simulink model "magDesat_test_2"  (R2018b)
settings: Solver=FixedStepAuto  StartTime=0.0  StopTime=25000  RelTol=1e-3
undefined symbols (not defined in the file or in its folder): DiscIntNeverNeededParam, fswParams, satelliteDynamics_lib, simParams
libraries: vrlib x2, Desaturation_Controller_lib x1, Detumbling_Controller_lib x1, Environment_lib x1, rwa_assembly_torqueinput_lib x1, aerolibutil x1, sharedutil x1
settings Model: Creator=colem  LastModifiedBy=colem

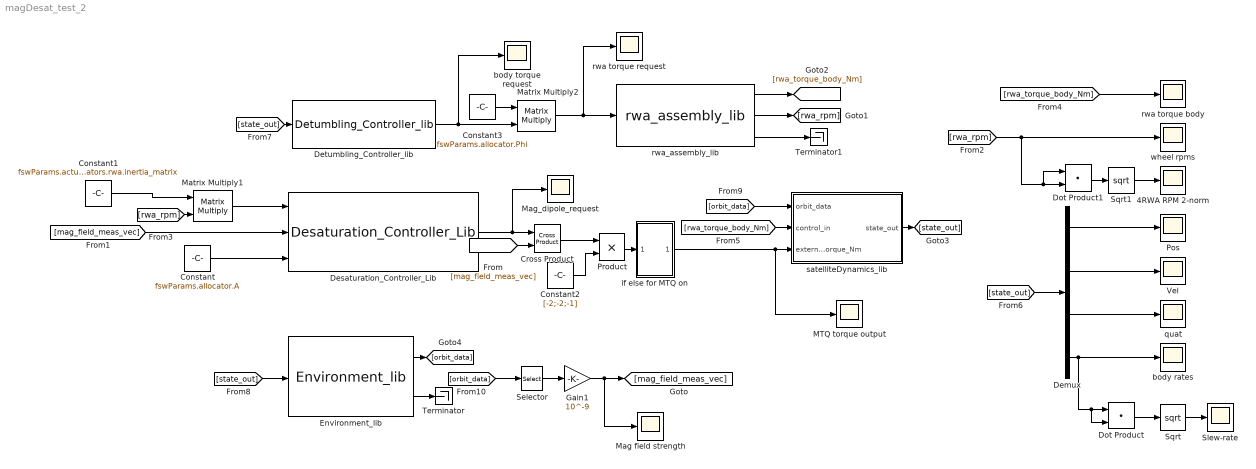
== system magDesat_test_2 ==
  4RWA RPM 2-norm : Scope
  Constant : Constant  Value=fswParams.allocator.A
  Constant1 : Constant  Value=fswParams.actuators.rwa.inertia_matrix
  Constant2 : Constant  Value=[-2;-2;-1]
  Constant3 : Constant  Value=fswParams.allocator.Phi
  Cross Product : vrlib/Utilities/Cross Product
      settings: SourceProductBaseCode=VR
  Demux : Demux  Outputs=[3 3 4 3]
  Desaturation_Controller_Lib : Desaturation_Controller_lib/Desaturation_Controller_Lib  SystemSampleTime=-1
  Detumbling_Controller_lib : Detumbling_Controller_lib/Detumbling_Controller_lib  SystemSampleTime=-1
  Dot Product : DotProduct  InputSameDT=on  OutDataTypeStr=Inherit: Inherit via internal rule
  Dot Product1 : DotProduct  InputSameDT=on  OutDataTypeStr=Inherit: Inherit via internal rule
  Environment_lib : Environment_lib/Environment_lib  SystemSampleTime=-1
  Gain1 : Gain  Gain=10^-9
  MTQ torque output : Scope
  Mag field strength : Scope
  Mag_dipole_request : Scope
  Matrix Multiply1 : Product  Multiplication=Matrix(*)
  Matrix Multiply2 : Product  Multiplication=Matrix(*)
  Pos : Scope
  Product : Product
  Selector : Selector  InputPortWidth=13  IndexOptions=Index vector (dialog)  Indices=[11 12 13]  OutputSizes=1
  Slew-rate : Scope
  Sqrt : Sqrt  SaturateOnIntegerOverflow=on
  Sqrt1 : Sqrt  SaturateOnIntegerOverflow=on
  Terminator : Terminator
  Terminator1 : Terminator
  Vel : Scope
  body rates : Scope
  body torque request : Scope
  if else for MTQ on : Subsystem
  quat : Scope
  rwa torque body : Scope
  rwa torque request : Scope
  rwa_assembly_lib : rwa_assembly_torqueinput_lib/rwa_assembly_lib  SystemSampleTime=-1
  satelliteDynamics_lib : Subsystem  AncestorBlock=satelliteDynamics_lib/satelliteDynamics_lib
  wheel rpms : Scope
  wires:
  Detumbling_Controller_lib/1 -> Matrix Multiply2/2, body torque request/1
  Environment_lib/2 -> Terminator/1
  Desaturation_Controller_Lib/1 -> Mag_dipole_request/1, Cross Product/1
  Constant/1 -> Desaturation_Controller_Lib/3
  Cross Product/1 -> Product/1
  Constant1/1 -> Matrix Multiply1/1
  rwa_assembly_lib/3 -> Terminator1/1
  Matrix Multiply1/1 -> Desaturation_Controller_Lib/1
  Constant3/1 -> Matrix Multiply2/1
  Matrix Multiply2/1 -> rwa_assembly_lib/1, rwa torque request/1
  [mag_field_meas_vec] -> Desaturation_Controller_Lib/2
  [mag_field_meas_vec] -> Cross Product/2
  Product/1 -> if else for MTQ on/1(In1)
  if else for MTQ on/1(Out1) -> MTQ torque output/1, satelliteDynamics_lib/3(external_torque_Nm)
  Selector/1 -> Gain1/1
  Gain1/1 -> Mag field strength/1, [mag_field_meas_vec]
  Dot Product/1 -> Sqrt/1
  Sqrt/1 -> Slew-rate/1
  Sqrt1/1 -> 4RWA RPM 2-norm/1
  Dot Product1/1 -> Sqrt1/1
  Demux/4 -> Dot Product/1, Dot Product/2, body rates/1
  Demux/3 -> quat/1
  Demux/2 -> Vel/1
  Demux/1 -> Pos/1
  Constant2/1 -> Product/2
  [rwa_rpm] -> Matrix Multiply1/2
  rwa_assembly_lib/2 -> [rwa_rpm]
  [rwa_rpm] -> wheel rpms/1, Dot Product1/1, Dot Product1/2
  [rwa_torque_body_Nm] -> satelliteDynamics_lib/2(control_in)
  [rwa_torque_body_Nm] -> rwa torque body/1
  rwa_assembly_lib/1 -> [rwa_torque_body_Nm]
  satelliteDynamics_lib/1(state_out) -> [state_out]
  [state_out] -> Demux/1
  [state_out] -> Environment_lib/1
  [state_out] -> Detumbling_Controller_lib/1
  [orbit_data] -> Selector/1
  [orbit_data] -> satelliteDynamics_lib/1(orbit_data)
  Environment_lib/1 -> [orbit_data]

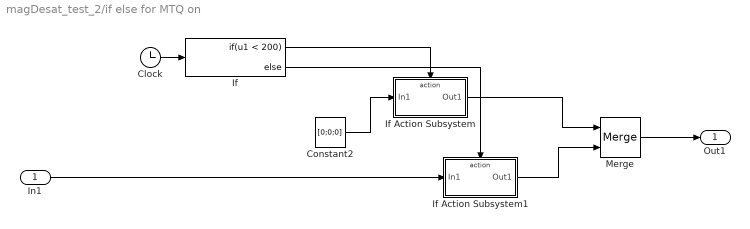
== system magDesat_test_2/if else for MTQ on ==
  In1 : Inport
  Clock : Clock
  Constant2 : Constant  Value=[0;0;0]
  If : If  IfExpression=u1 < 200
  If Action Subsystem : Subsystem  TreatAsAtomicUnit=on
  If Action Subsystem1 : Subsystem  TreatAsAtomicUnit=on
  Merge : Merge
  Out1 : Outport
  wires:
  Clock/1 -> If/1
  If/2 -> If Action Subsystem1/Action
  Constant2/1 -> If Action Subsystem/1(In1)
  Merge/1 -> Out1/1
  If Action Subsystem1/1(Out1) -> Merge/2
  If Action Subsystem/1(Out1) -> Merge/1
  If/1 -> If Action Subsystem/Action
  In1/1 -> If Action Subsystem1/1(In1)

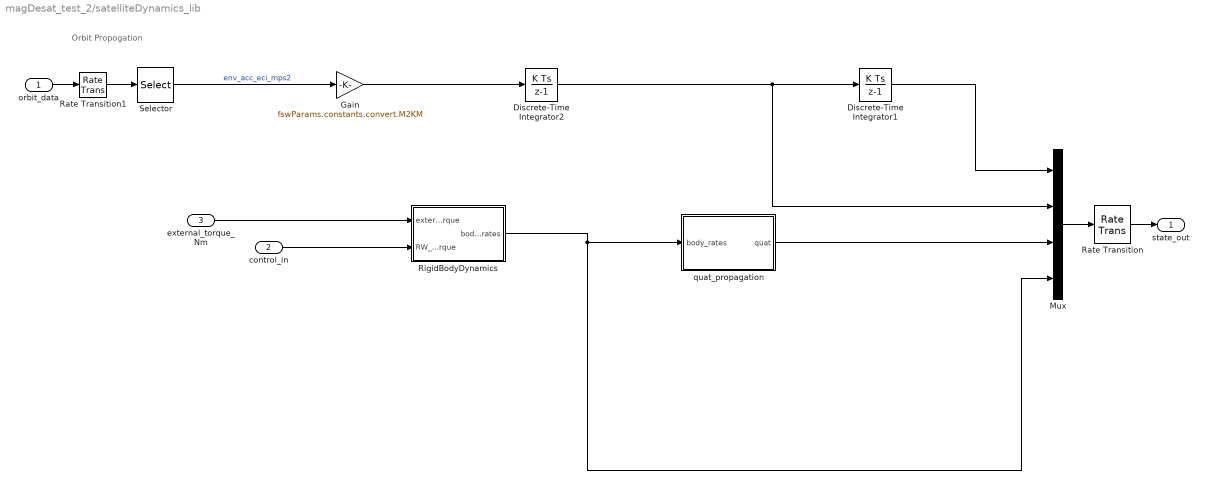
== system magDesat_test_2/satelliteDynamics_lib ==
  note: Orbit Propogation
  orbit_data : Inport
  control_in : Inport  Port=2
  external_torque_Nm : Inport  Port=3
  Discrete-Time Integrator1 : DiscreteIntegrator  InitialCondition=simParams.initialConditions.r0  SampleTime=-1  ICPrevOutput=DiscIntNeverNeededParam  ICPrevScaledInput=DiscIntNeverNeededParam
  Discrete-Time Integrator2 : DiscreteIntegrator  InitialCondition=simParams.initialConditions.v0  SampleTime=-1  ICPrevOutput=DiscIntNeverNeededParam  ICPrevScaledInput=DiscIntNeverNeededParam
  Gain : Gain  Gain=fswParams.constants.convert.M2KM
  Mux : Mux  Inputs=[3 3 4 3]
  Rate Transition : RateTransition  InitialCondition=[simParams.initialConditions.r0;simParams.initialConditions.v0;simParams.initialConditions.q0;simParams.initialConditions.w0]
  Rate Transition1 : RateTransition  OutPortSampleTime=simParams.sample_time_s
  RigidBodyDynamics : Subsystem
  Selector : Selector  InputPortWidth=13  IndexOptions=Index vector (dialog)  Indices=[1 2 3]  OutputSizes=1
  quat_propagation : Subsystem
  state_out : Outport
  wires:
  control_in/1 -> RigidBodyDynamics/2(RW_torque)
  Mux/1 -> Rate Transition/1
  Discrete-Time Integrator2/1 -> Mux/2, Discrete-Time Integrator1/1
  Discrete-Time Integrator1/1 -> Mux/1
  Gain/1 -> Discrete-Time Integrator2/1
  Rate Transition/1 -> state_out/1
  orbit_data/1 -> Rate Transition1/1
  Rate Transition1/1 -> Selector/1
  external_torque_Nm/1 -> RigidBodyDynamics/1(external_torque)
  Selector/1 -> Gain/1  "env_acc_eci_mps2"
  quat_propagation/1(quat) -> Mux/3
  RigidBodyDynamics/1(body_rates) -> Mux/4, quat_propagation/1(body_rates)

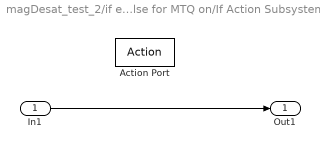
== system magDesat_test_2/if else for MTQ on/If Action Subsystem ==
  In1 : Inport
  Action Port : ActionPort  ActionType=then
  Out1 : Outport
  wires:
  In1/1 -> Out1/1

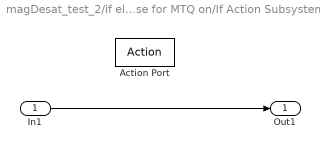
== system magDesat_test_2/if else for MTQ on/If Action Subsystem1 ==
  In1 : Inport
  Action Port : ActionPort  ActionType=else
  Out1 : Outport
  wires:
  In1/1 -> Out1/1

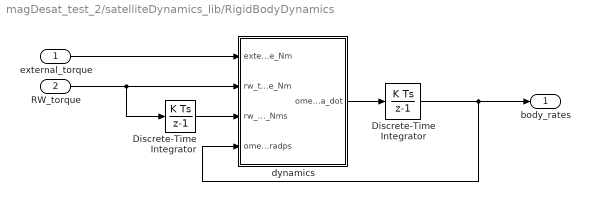
== system magDesat_test_2/satelliteDynamics_lib/RigidBodyDynamics ==
  external_torque : Inport
  RW_torque : Inport  Port=2
  Discrete-Time Integrator : DiscreteIntegrator  InitialCondition=[0;0;0]  SampleTime=-1  ICPrevOutput=DiscIntNeverNeededParam  ICPrevScaledInput=DiscIntNeverNeededParam
  "Discrete-Time Integrator " : DiscreteIntegrator  InitialCondition=simParams.initialConditions.w0  SampleTime=-1  ICPrevOutput=DiscIntNeverNeededParam  ICPrevScaledInput=DiscIntNeverNeededParam
  dynamics : Subsystem
  body_rates : Outport
  wires:
  RW_torque/1 -> dynamics/2(rw_torque_Nm), Discrete-Time Integrator/1
  Discrete-Time Integrator/1 -> dynamics/3(rw_momentum_Nms)
  "Discrete-Time Integrator "/1 -> body_rates/1, dynamics/4(omega_radps)
  external_torque/1 -> dynamics/1(external_torque_Nm)
  dynamics/1(omega_dot) -> "Discrete-Time Integrator "/1

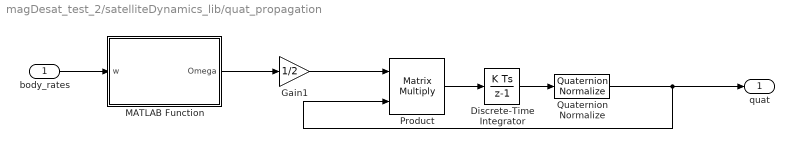
== system magDesat_test_2/satelliteDynamics_lib/quat_propagation ==
  body_rates : Inport
  Discrete-Time Integrator : DiscreteIntegrator  InitialCondition=simParams.initialConditions.q0  SampleTime=-1  ICPrevOutput=DiscIntNeverNeededParam  ICPrevScaledInput=DiscIntNeverNeededParam
  Gain1 : Gain  Gain=1/2
  MATLAB Function : MATLAB Function  TreatAsAtomicUnit=on
  Product : Product  Multiplication=Matrix(*)  RndMeth=Zero
  Quaternion Normalize : sharedutil/Quaternion Normalize  aMode=aMode
      settings: SourceProductName=Aerospace Blockset  SourceProductBaseCode=AE
  quat : Outport
  wires:
  Product/1 -> Discrete-Time Integrator/1
  Discrete-Time Integrator/1 -> Quaternion Normalize/1
  Gain1/1 -> Product/1
  Quaternion Normalize/1 -> quat/1, Product/2
  body_rates/1 -> MATLAB Function/1(w)
  MATLAB Function/1(Omega) -> Gain1/1

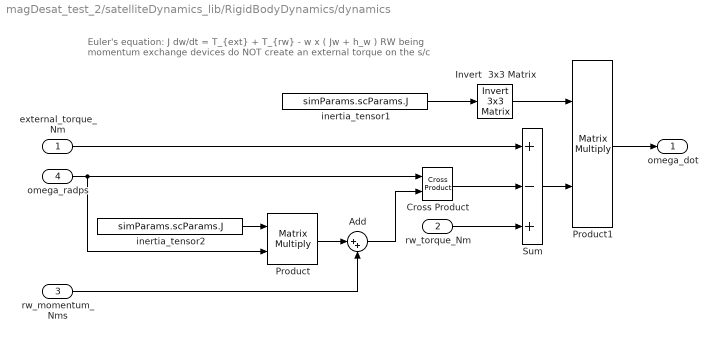
== system magDesat_test_2/satelliteDynamics_lib/RigidBodyDynamics/dynamics ==
  note: Euler's equation: J dw/dt = T_{ext} + T_{rw} - w x ( Jw + h_w )
      |
      | RW being momentum exchange devices do NOT create
      | an external torque on the s/c
  external_torque_Nm : Inport
  rw_torque_Nm : Inport  Port=2
  rw_momentum_Nms : Inport  Port=3
  omega_radps : Inport  Port=4
  Add : Sum  Inputs=|++
  Cross Product : vrlib/Utilities/Cross Product
      settings: SourceProductBaseCode=VR
  Invert  3x3 Matrix : aerolibutil/Invert  3x3 Matrix
  Product : Product  Multiplication=Matrix(*)  RndMeth=Zero
  Product1 : Product  Multiplication=Matrix(*)  RndMeth=Zero
  Sum : Sum  Inputs=+-+
  inertia_tensor1 : Constant  Value=simParams.scParams.J  SampleTime=simParams.sample_time_s
  inertia_tensor2 : Constant  Value=simParams.scParams.J  SampleTime=simParams.sample_time_s
  omega_dot : Outport
  wires:
  rw_torque_Nm/1 -> Sum/3
  Add/1 -> Cross Product/2
  Product/1 -> Add/1
  Cross Product/1 -> Sum/2
  inertia_tensor1/1 -> Invert  3x3 Matrix/1
  Invert  3x3 Matrix/1 -> Product1/1
  Product1/1 -> omega_dot/1
  Sum/1 -> Product1/2
  inertia_tensor2/1 -> Product/1
  omega_radps/1 -> Cross Product/1, Product/2
  external_torque_Nm/1 -> Sum/1
  rw_momentum_Nms/1 -> Add/2

== matlab function magDesat_test_2/satelliteDynamics_lib/quat_propagation/MATLAB Function ==
  data: w input; Omega output
function Omega = skew_sym(w)
%#codegen

    w_skew = ...
        [0 w(3) -w(2);
        -w(3) 0 w(1);
        w(2) -w(1) 0];

    Omega = ...
        [0 -w';
        w w_skew];
